simulink model "GunControllerMega"  (R2020a)
settings: Solver=FixedStepAuto  StartTime=0.0  StopTime=inf  FixedStep=0.025  RelTol=1e-3  EnableMultiTasking=on
model workspace (MAT data in the model file):
  RadioAnalogByteTwo = 204
values from neighbouring files (symbols this model uses):
  CANok = 0    [Parameters.m]
  RadioAnalogByteFive = 51    [Parameters.m]
  RadioAnalogByteFour = 51    [Parameters.m]
  RadioAnalogByteOne = 87.140625    [Parameters.m]
  RadioAnalogByteSeven = 51    [Parameters.m]
  RadioAnalogByteSix = 51    [Parameters.m]
  RadioAnalogByteThree = 51    [Parameters.m]
  RadioAnalogByteZero = 51    [Parameters.m]
libraries: ScaleOneEighty x8, arduinolib x7, simulink x6
settings Model: SILPILModeSetting=veronly  ExtModeTrigDuration=2  Creator=marqu  LastModifiedBy=marqu
settings OptimizationCC: EnhancedBackFolding=on  PassReuseOutputArgsAs=Individual arguments  ZeroExternalMemoryAtStartup=off  ZeroInternalMemoryAtStartup=off  MaxStackSize=64  OptimizeBlockOrder=speed  DifferentSizesBufferReuse=on  OptimizationCustomize=off  EfficientTunableParamExpr=on
settings DebuggingCC: ParameterTunabilityLossMsg=error
settings HardwareCC: ProdBitPerInt=16  ProdBitPerPointer=16  ProdBitPerSizeT=16  ProdBitPerPtrDiffT=16  ProdLargestAtomicFloat=None  ProdWordSize=8  ProdHWDeviceType=Atmel->AVR  UseEmbeddedCoderFeatures=off  UseSimulinkCoderFeatures=off
settings SFSimCC: MATLABDynamicMemAlloc=off
settings RTWCC: SystemTargetFile=ert.tlc  HardwareBoard=Arduino Mega 2560  TLCOptions=-aInlineSetEventsForThisBaseRateFcn=TLC_FALSE -aSuppressMultiTaskScheduler=TLC_FALSE -aRateBasedStepFcn=1  TemplateMakefile=ert_default_tmf  Toolchain=Arduino AVR  BuildConfiguration=Faster Runs
settings CodeAppCC: ForceParamTrailComments=on  IgnoreCustomStorageClasses=off  OperatorAnnotations=on  SimulinkDataObjDesc=on  SFDataObjDesc=on  InsertBlockDesc=on
settings ERTTargetCC: SupportContinuousTime=on  SupportNonInlinedSFcns=on  SupportVariableSizeSignals=on  ExtModeStaticAllocSize=2048

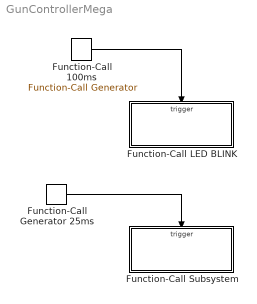
== system GunControllerMega ==
  Function-Call 100ms : simulink/Ports & Subsystems/Function-Call Generator  sample_time=0.1  numberOfIterations=1
  Function-Call Generator 25ms : simulink/Ports & Subsystems/Function-Call Generator  sample_time=0.025  numberOfIterations=1
  Function-Call Subsystem : Subsystem  TreatAsAtomicUnit=on
  Function-Call LED BLINK : Subsystem  TreatAsAtomicUnit=on
  wires:
  Function-Call Generator 25ms/1 -> Function-Call Subsystem/Trigger
  Function-Call 100ms/1 -> Function-Call LED BLINK/Trigger

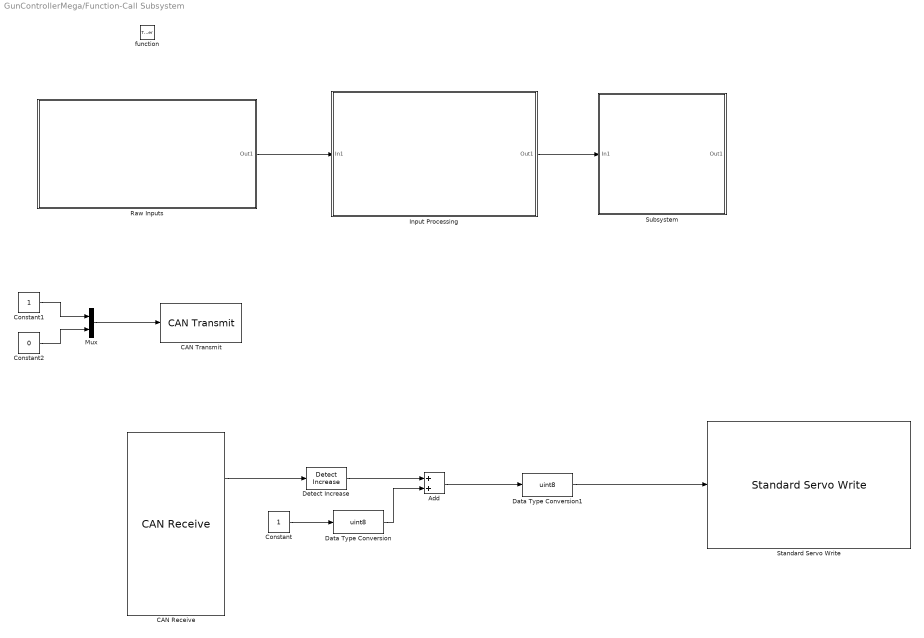
== system GunControllerMega/Function-Call Subsystem ==
  function : TriggerPort  TriggerType=function-call  VariantControl=Variant
  Add : Sum
  CAN Receive : arduinolib/CAN Receive  outputDataType=Raw data  identifierType=Standard (11-bit identifier)  messageId=512  msgLength=1  SampleTime=inf  outputError=off  outputRemote=off
      settings: SourceProductBaseCode=ARDUINO
  CAN Transmit : arduinolib/CAN Transmit  inputDataType=Raw data  BlockingMode_=off  BlockTimeout_=1  outputStatus=off  identifierType=Standard (11-bit identifier)  messageId=22  msgLength=2  remoteFrame=off
      settings: SourceProductBaseCode=ARDUINO
  Constant : Constant
  Constant1 : Constant  OutDataTypeStr=uint8
  Constant2 : Constant  Value=0  OutDataTypeStr=uint8
  Data Type Conversion : DataTypeConversion  OutDataTypeStr=uint8
  Data Type Conversion1 : DataTypeConversion  OutDataTypeStr=uint8
  Detect Increase : simulink/Logic and Bit Operations/Detect Increase  vinit=0.0  OutDataTypeStr=boolean
  "Input Processing " : Subsystem
  Mux : Mux  Inputs=2
  Raw Inputs : Subsystem
  Standard Servo Write : arduinolib/Standard Servo Write  pinNumber=11  ServoIndex=0  blockPlatform=ARDUINO
  Subsystem : Subsystem
  wires:
  Constant1/1 -> Mux/1
  Mux/1 -> CAN Transmit/1
  Constant2/1 -> Mux/2
  Raw Inputs/1(Out1) -> "Input Processing "/1(In1)
  "Input Processing "/1(Out1) -> Subsystem/1(In1)
  CAN Receive/1 -> Detect Increase/1
  Add/1 -> Data Type Conversion1/1
  Constant/1 -> Data Type Conversion/1
  Data Type Conversion/1 -> Add/2
  Data Type Conversion1/1 -> Standard Servo Write/1
  Detect Increase/1 -> Add/1

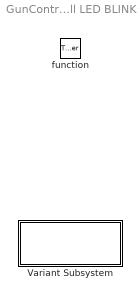
== system GunControllerMega/Function-Call LED BLINK ==
  function : TriggerPort  TriggerType=function-call  VariantControl=Variant
  Variant Subsystem : Subsystem  Variant=on

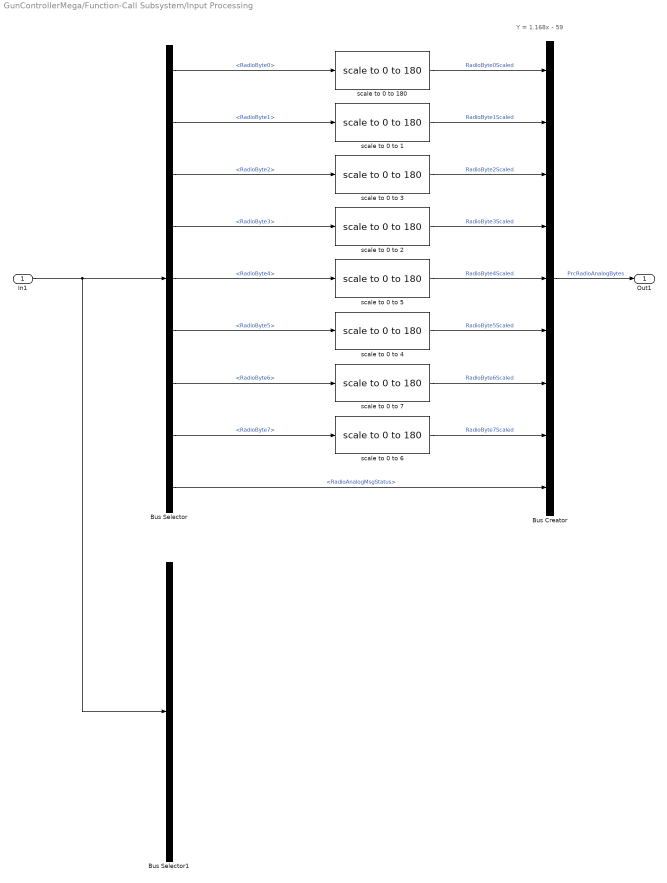
== system GunControllerMega/Function-Call Subsystem/Input Processing  ==
  note: Y = 1.168x - 59
  In1 : Inport
  Bus Creator : BusCreator  Inputs=9
  Bus Selector : BusSelector  OutputSignals=RadioAnalogMsg.RadioByte0,RadioAnalogMsg.RadioByte1,RadioAnalogMsg.RadioByte2,RadioAnalogMsg.RadioByte3,RadioAnalogMsg.RadioByte4,RadioAnalogMsg.RadioByte5,RadioAnalogMsg.RadioByte6,RadioAnalogMsg.RadioByte7,RadioAnalogMsg.RadioAnalogMsgStatus
  Bus Selector1 : BusSelector  OutputSignals=RadioDigitalMsg.RadioDigByte0,RadioDigitalMsg.RadioDigByte1,RadioDigitalMsg.RadioDigByte2,RadioDigitalMsg.RadioDigByte3,RadioDigitalMsg.RadioDigByte4,RadioDigitalMsg.RadioDigByte5,RadioDigitalMsg.RadioDigByte6,RadioDigitalMsg.RadioDigByte7,RadioDigitalMsg.RadioDigitalMsgStatus
  scale to 0 to {1..7,180} (8 alike) : ScaleOneEighty/scale to 0 to 180  SystemSampleTime=-1  Latency=0  AutoFrameSizeCalculation=off
  Out1 : Outport
  wires:
  Bus Selector/6 -> scale to 0 to 4/1  "<RadioByte5>"
  In1/1 -> Bus Selector1/1, Bus Selector/1
  Bus Selector/5 -> scale to 0 to 5/1  "<RadioByte4>"
  Bus Selector/4 -> scale to 0 to 2/1  "<RadioByte3>"
  Bus Selector/8 -> scale to 0 to 6/1  "<RadioByte7>"
  Bus Selector/2 -> scale to 0 to 1/1  "<RadioByte1>"
  Bus Selector/3 -> scale to 0 to 3/1  "<RadioByte2>"
  Bus Selector/1 -> scale to 0 to 180/1  "<RadioByte0>"
  Bus Selector/7 -> scale to 0 to 7/1  "<RadioByte6>"
  scale to 0 to 180/1 -> Bus Creator/1  "RadioByte0Scaled"
  scale to 0 to 1/1 -> Bus Creator/2  "RadioByte1Scaled"
  scale to 0 to 3/1 -> Bus Creator/3  "RadioByte2Scaled"
  Bus Selector/9 -> Bus Creator/9  "<RadioAnalogMsgStatus>"
  scale to 0 to 6/1 -> Bus Creator/8  "RadioByte7Scaled"
  scale to 0 to 7/1 -> Bus Creator/7  "RadioByte6Scaled"
  scale to 0 to 4/1 -> Bus Creator/6  "RadioByte5Scaled"
  scale to 0 to 5/1 -> Bus Creator/5  "RadioByte4Scaled"
  scale to 0 to 2/1 -> Bus Creator/4  "RadioByte3Scaled"
  Bus Creator/1 -> Out1/1  "PrcRadioAnalogBytes"

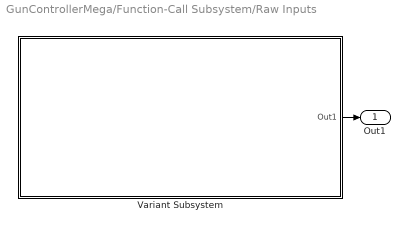
== system GunControllerMega/Function-Call Subsystem/Raw Inputs ==
  Variant Subsystem : Subsystem  Variant=on
  Out1 : Outport
  wires:
  Variant Subsystem/1(Out1) -> Out1/1

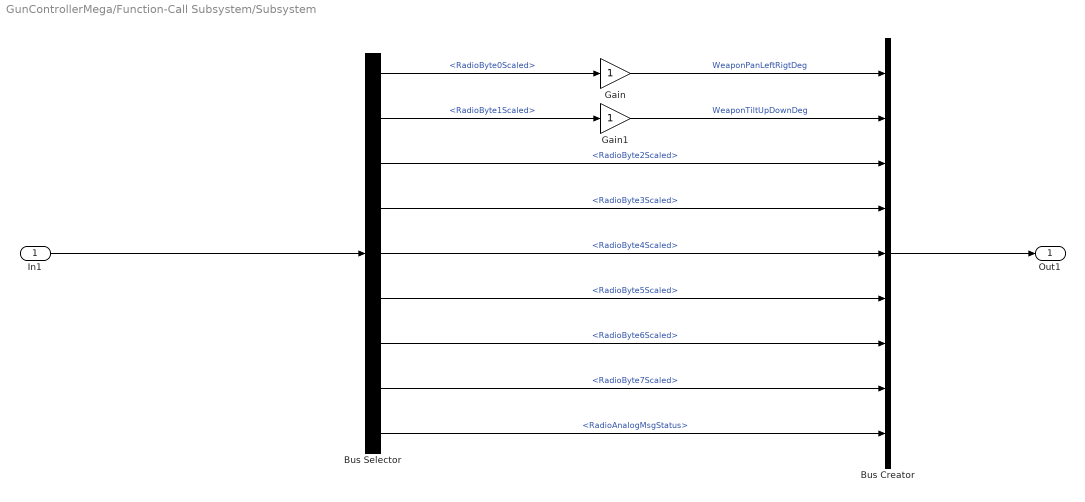
== system GunControllerMega/Function-Call Subsystem/Subsystem ==
  In1 : Inport
  Bus Creator : BusCreator  Inputs=9
  Bus Selector : BusSelector  OutputSignals=RadioByte0Scaled,RadioByte1Scaled,RadioByte2Scaled,RadioByte3Scaled,RadioByte4Scaled,RadioByte5Scaled,RadioByte6Scaled,RadioByte7Scaled,RadioAnalogMsgStatus
  Gain : Gain  OutDataTypeStr=uint8
  Gain1 : Gain  OutDataTypeStr=uint8
  Out1 : Outport
  wires:
  Bus Selector/2 -> Gain1/1  "<RadioByte1Scaled>"
  In1/1 -> Bus Selector/1
  Bus Selector/1 -> Gain/1  "<RadioByte0Scaled>"
  Bus Selector/3 -> Bus Creator/3  "<RadioByte2Scaled>"
  Bus Selector/4 -> Bus Creator/4  "<RadioByte3Scaled>"
  Gain/1 -> Bus Creator/1  "WeaponPanLeftRigtDeg"
  Gain1/1 -> Bus Creator/2  "WeaponTiltUpDownDeg"
  Bus Selector/5 -> Bus Creator/5  "<RadioByte4Scaled>"
  Bus Selector/9 -> Bus Creator/9  "<RadioAnalogMsgStatus>"
  Bus Selector/8 -> Bus Creator/8  "<RadioByte7Scaled>"
  Bus Selector/6 -> Bus Creator/6  "<RadioByte5Scaled>"
  Bus Selector/7 -> Bus Creator/7  "<RadioByte6Scaled>"
  Bus Creator/1 -> Out1/1

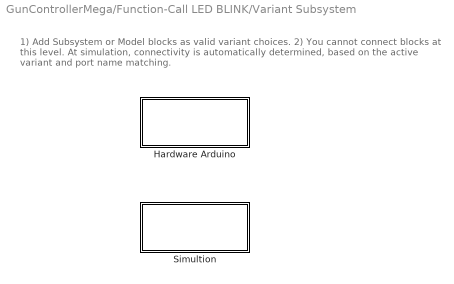
== system GunControllerMega/Function-Call LED BLINK/Variant Subsystem ==
  note: 1) Add Subsystem or Model blocks as valid variant choices.
      | 2) You cannot connect blocks at this level. At simulation, connectivity is automatically
      | determined, based on the active variant and port name matching.
  Hardware Arduino : Subsystem  VariantControl=(default)
  Simultion : Subsystem  VariantControl=Choice_2

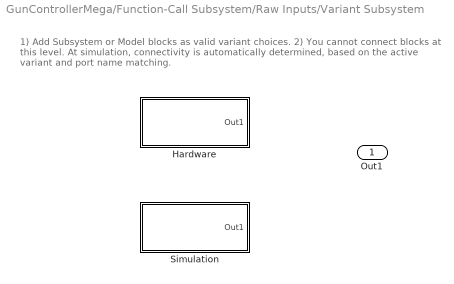
== system GunControllerMega/Function-Call Subsystem/Raw Inputs/Variant Subsystem ==
  note: 1) Add Subsystem or Model blocks as valid variant choices.
      | 2) You cannot connect blocks at this level. At simulation, connectivity is automatically
      | determined, based on the active variant and port name matching.
  Hardware : Subsystem  VariantControl=(default)
  "Simulation " : Subsystem  VariantControl=Choice_2
  Out1 : Outport

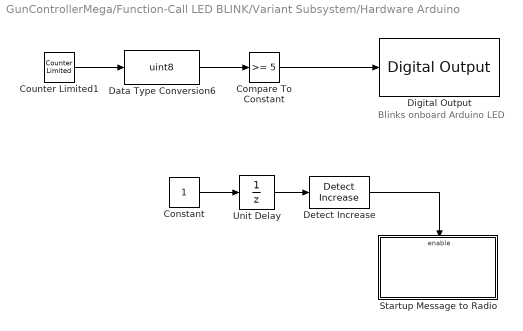
== system GunControllerMega/Function-Call LED BLINK/Variant Subsystem/Hardware Arduino ==
  note: Blinks onboard Arduino LED
  Compare To Constant : simulink/Logic and Bit Operations/Compare To Constant  relop=>=  const=5  OutDataTypeStr=boolean
  Constant : Constant  OutDataTypeStr=boolean
  Counter Limited1 : simulink/Sources/Counter Limited  uplimit=10  tsamp=-1
  Data Type Conversion6 : DataTypeConversion  OutDataTypeStr=uint8
  Detect Increase : simulink/Logic and Bit Operations/Detect Increase  vinit=0.0  OutDataTypeStr=boolean
  Digital Output : arduinolib/Digital Output  pinNumber=13  Direction=output  blockPlatform=arduino
  Startup Message to Radio : Subsystem
  Unit Delay : UnitDelay  SampleTime=-1  HasFrameUpgradeWarning=on
  wires:
  Counter Limited1/1 -> Data Type Conversion6/1
  Detect Increase/1 -> Startup Message to Radio/Enable
  Constant/1 -> Unit Delay/1
  Unit Delay/1 -> Detect Increase/1
  Compare To Constant/1 -> Digital Output/1
  Data Type Conversion6/1 -> Compare To Constant/1

== system GunControllerMega/Function-Call LED BLINK/Variant Subsystem/Simultion ==

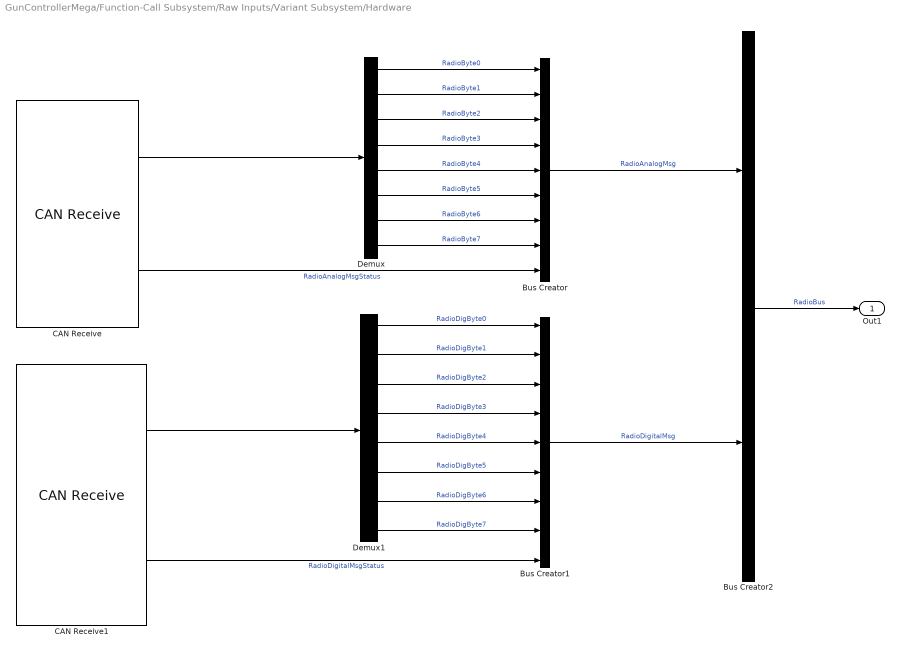
== system GunControllerMega/Function-Call Subsystem/Raw Inputs/Variant Subsystem/Hardware ==
  Bus Creator : BusCreator  Inputs=9
  Bus Creator1 : BusCreator  Inputs=9
  Bus Creator2 : BusCreator  Inputs=2
  CAN Receive : arduinolib/CAN Receive  outputDataType=Raw data  identifierType=Standard (11-bit identifier)  messageId=484  msgLength=8  SampleTime=inf  outputError=off  outputRemote=off
      settings: SourceProductBaseCode=ARDUINO
  CAN Receive1 : arduinolib/CAN Receive  outputDataType=Raw data  identifierType=Standard (11-bit identifier)  messageId=740  msgLength=8  SampleTime=inf  outputError=off  outputRemote=off
      settings: SourceProductBaseCode=ARDUINO
  Demux : Demux  Outputs=8
  Demux1 : Demux  Outputs=8
  Out1 : Outport
  wires:
  CAN Receive/1 -> Demux/1
  Demux/1 -> Bus Creator/1  "RadioByte0"
  Demux/2 -> Bus Creator/2  "RadioByte1"
  Demux/3 -> Bus Creator/3  "RadioByte2"
  Demux/4 -> Bus Creator/4  "RadioByte3"
  Demux/5 -> Bus Creator/5  "RadioByte4"
  Demux/6 -> Bus Creator/6  "RadioByte5"
  Demux/7 -> Bus Creator/7  "RadioByte6"
  Demux/8 -> Bus Creator/8  "RadioByte7"
  Bus Creator/1 -> Bus Creator2/1  "RadioAnalogMsg"
  CAN Receive/2 -> Bus Creator/9  "RadioAnalogMsgStatus"
  CAN Receive1/1 -> Demux1/1
  Demux1/8 -> Bus Creator1/8  "RadioDigByte7"
  Demux1/1 -> Bus Creator1/1  "RadioDigByte0"
  Demux1/2 -> Bus Creator1/2  "RadioDigByte1"
  Demux1/3 -> Bus Creator1/3  "RadioDigByte2"
  Demux1/4 -> Bus Creator1/4  "RadioDigByte3"
  Demux1/5 -> Bus Creator1/5  "RadioDigByte4"
  Demux1/6 -> Bus Creator1/6  "RadioDigByte5"
  Demux1/7 -> Bus Creator1/7  "RadioDigByte6"
  CAN Receive1/2 -> Bus Creator1/9  "RadioDigitalMsgStatus"
  Bus Creator1/1 -> Bus Creator2/2  "RadioDigitalMsg"
  Bus Creator2/1 -> Out1/1  "RadioBus"

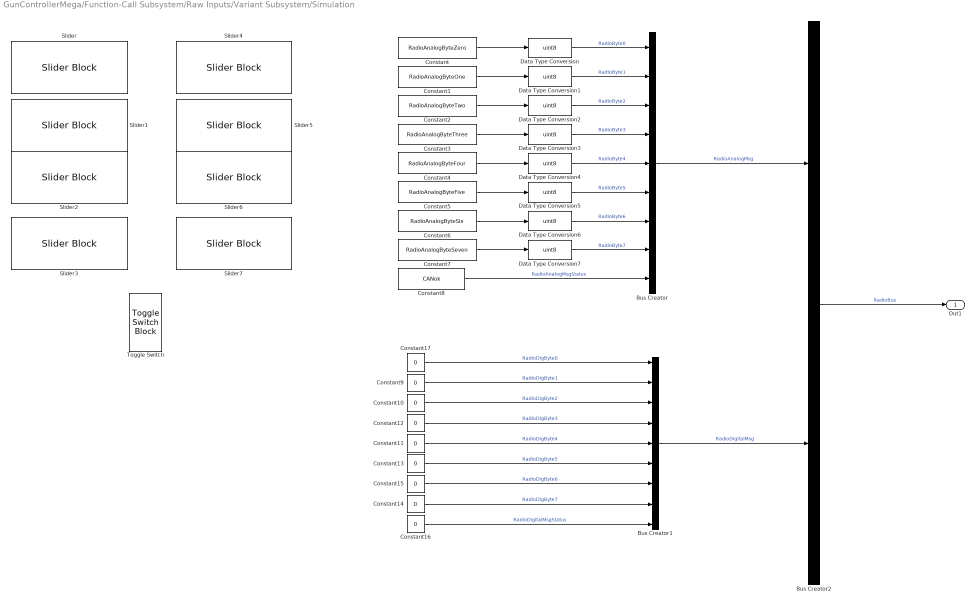
== system GunControllerMega/Function-Call Subsystem/Raw Inputs/Variant Subsystem/Simulation  ==
  Bus Creator : BusCreator  Inputs=9
  Bus Creator1 : BusCreator  Inputs=9
  Bus Creator2 : BusCreator  Inputs=2
  Constant : Constant  Value=RadioAnalogByteZero
  Constant1 : Constant  Value=RadioAnalogByteOne
  Constant{9..17} (9 alike) : Constant  Value=0  OutDataTypeStr=uint8
  Constant2 : Constant  Value=RadioAnalogByteTwo
  Constant3 : Constant  Value=RadioAnalogByteThree
  Constant4 : Constant  Value=RadioAnalogByteFour
  Constant5 : Constant  Value=RadioAnalogByteFive
  Constant6 : Constant  Value=RadioAnalogByteSix
  Constant7 : Constant  Value=RadioAnalogByteSeven
  Constant8 : Constant  Value=CANok  OutDataTypeStr=uint8  SampleTime=-1
  Data Type Conversion{,1..7} (8 alike) : DataTypeConversion  OutDataTypeStr=uint8
  Slider : SliderBlock  ScaleMin=51  ScaleMax=201
  Slider{1..7} (7 alike) : SliderBlock  ScaleMin=51  ScaleMax=204
  Toggle Switch : ToggleSwitchBlock
      settings: Values={{'Off', 'On'}, [0 1]}
  Out1 : Outport
  wires:
  Constant8/1 -> Bus Creator/9  "RadioAnalogMsgStatus"
  Constant7/1 -> Data Type Conversion7/1
  Constant1/1 -> Data Type Conversion1/1
  Constant5/1 -> Data Type Conversion5/1
  Constant/1 -> Data Type Conversion/1
  Constant3/1 -> Data Type Conversion3/1
  Constant2/1 -> Data Type Conversion2/1
  Constant4/1 -> Data Type Conversion4/1
  Constant6/1 -> Data Type Conversion6/1
  Bus Creator/1 -> Bus Creator2/1  "RadioAnalogMsg"
  Data Type Conversion/1 -> Bus Creator/1  "RadioByte0"
  Data Type Conversion1/1 -> Bus Creator/2  "RadioByte1"
  Data Type Conversion2/1 -> Bus Creator/3  "RadioByte2"
  Data Type Conversion3/1 -> Bus Creator/4  "RadioByte3"
  Data Type Conversion6/1 -> Bus Creator/7  "RadioByte6"
  Data Type Conversion4/1 -> Bus Creator/5  "RadioByte4"
  Data Type Conversion5/1 -> Bus Creator/6  "RadioByte5"
  Data Type Conversion7/1 -> Bus Creator/8  "RadioByte7"
  Constant10/1 -> Bus Creator1/3  "RadioDigByte2"
  Constant12/1 -> Bus Creator1/4  "RadioDigByte3"
  Constant9/1 -> Bus Creator1/2  "RadioDigByte1"
  Constant14/1 -> Bus Creator1/8  "RadioDigByte7"
  Constant16/1 -> Bus Creator1/9  "RadioDigitalMsgStatus"
  Constant15/1 -> Bus Creator1/7  "RadioDigByte6"
  Constant13/1 -> Bus Creator1/6  "RadioDigByte5"
  Constant11/1 -> Bus Creator1/5  "RadioDigByte4"
  Bus Creator1/1 -> Bus Creator2/2  "RadioDigitalMsg"
  Bus Creator2/1 -> Out1/1  "RadioBus"
  Constant17/1 -> Bus Creator1/1  "RadioDigByte0"

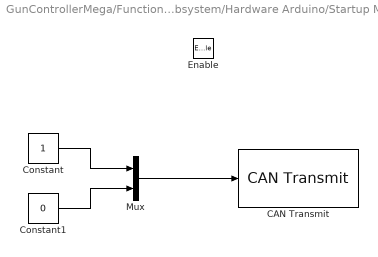
== system GunControllerMega/Function-Call LED BLINK/Variant Subsystem/Hardware Arduino/Startup Message to Radio ==
  Enable : EnablePort
  CAN Transmit : arduinolib/CAN Transmit  inputDataType=Raw data  BlockingMode_=off  BlockTimeout_=1  outputStatus=off  identifierType=Standard (11-bit identifier)  messageId=0  msgLength=2  remoteFrame=off
      settings: SourceProductBaseCode=ARDUINO
  Constant : Constant  OutDataTypeStr=uint8
  Constant1 : Constant  Value=0  OutDataTypeStr=uint8
  Mux : Mux  Inputs=2
  wires:
  Constant1/1 -> Mux/2
  Constant/1 -> Mux/1
  Mux/1 -> CAN Transmit/1
